simulink model "ASSIGNMENT1V6"  (R2020a)
settings: Solver=FixedStepAuto  StartTime=0.0  StopTime=5.0  FixedStep=1e-3  RelTol=1e-3  EnableMultiTasking=on
undefined symbols (not defined in the file): A0, A1, A3, A4, D0, D1, D10, D11, D12, D13, D2, D3, D4, D5, D6, D7, D8, D9, PTA0, PTA1, PTA2, PTB11, PTB2, PTB23, PTB3, PTB9, PTC11, PTC16, PTC17, PTC2, PTC3, PTC4, PTD0, PTD1, PTD2, PTD3
libraries: frdmk64flib x21
settings Model: ExtModeTrigDuration=5  Creator=Daniyal  LastModifiedBy=Daniyal
settings OptimizationCC: EnhancedBackFolding=on  PassReuseOutputArgsAs=Individual arguments  ZeroExternalMemoryAtStartup=off  ZeroInternalMemoryAtStartup=off  MaxStackSize=64  OptimizeBlockOrder=speed  DifferentSizesBufferReuse=on  OptimizationCustomize=off  EfficientTunableParamExpr=on
settings DebuggingCC: ParameterTunabilityLossMsg=error
settings HardwareCC: ProdBitPerPointer=32  ProdBitPerSizeT=32  ProdBitPerPtrDiffT=32  ProdLargestAtomicInteger=Long  ProdLargestAtomicFloat=Double  ProdWordSize=32  ProdHWDeviceType=ARM Compatible->ARM Cortex
settings SFSimCC: MATLABDynamicMemAlloc=off
settings RTWCC: SystemTargetFile=ert.tlc  HardwareBoard=NXP FRDM-K64F  TemplateMakefile=ert_default_tmf  Toolchain=GNU Tools for ARM Embedded Processors
settings CodeAppCC: ForceParamTrailComments=on  IgnoreCustomStorageClasses=off  OperatorAnnotations=on  SimulinkDataObjDesc=on  SFDataObjDesc=on  InsertBlockDesc=on

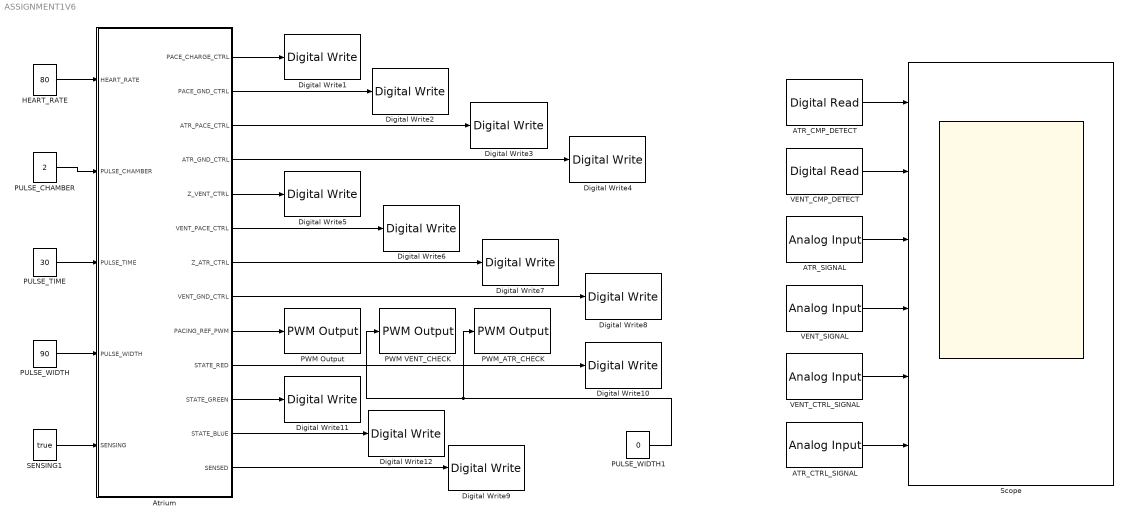
== system ASSIGNMENT1V6 ==
  ATR_CMP_DETECT : frdmk64flib/Digital Read  Whichpin=PTC16 (D0)  SampleTime=-1
  ATR_CTRL_SIGNAL : frdmk64flib/Analog Input  Whichpin=PTB11 (A3)  SampleTime=-1
  ATR_SIGNAL : frdmk64flib/Analog Input  Whichpin=PTB2 (A0)  SampleTime=-1
  Atrium : Stateflow chart  TreatAsAtomicUnit=on
  Digital Write1 : frdmk64flib/Digital Write  Whichpin=PTB9 (D2)
  Digital Write10 : frdmk64flib/Digital Write  Whichpin=RED_LED
  Digital Write11 : frdmk64flib/Digital Write  Whichpin=GREEN_LED
  Digital Write12 : frdmk64flib/Digital Write  Whichpin=BLUE_LED
  Digital Write2 : frdmk64flib/Digital Write  Whichpin=PTD0 (D10)
  Digital Write3 : frdmk64flib/Digital Write  Whichpin=PTA0 (D8)
  Digital Write4 : frdmk64flib/Digital Write  Whichpin=PTD2 (D11)
  Digital Write5 : frdmk64flib/Digital Write  Whichpin=PTC3 (D7)
  Digital Write6 : frdmk64flib/Digital Write  Whichpin=PTC4 (D9)
  Digital Write7 : frdmk64flib/Digital Write  Whichpin=PTB23 (D4)
  Digital Write8 : frdmk64flib/Digital Write  Whichpin=PTD3 (D12)
  Digital Write9 : frdmk64flib/Digital Write  Whichpin=PTD1 (D13)
  HEART_RATE : Constant  Value=80
  PULSE_CHAMBER : Constant  Value=2
  PULSE_TIME : Constant  Value=30
  PULSE_WIDTH : Constant  Value=90
  PULSE_WIDTH1 : Constant  Value=0
  PWM Output : frdmk64flib/PWM Output  Whichpin=PTA2 (D5)  InitialFrequency=2000  InitialDutyCycle=70
  PWM VENT_CHECK : frdmk64flib/PWM Output  Whichpin=PTA1 (D3)  InitialFrequency=2000  InitialDutyCycle=80
  PWM_ATR_CHECK : frdmk64flib/PWM Output  Whichpin=PTC2 (D6)  InitialFrequency=2000  InitialDutyCycle=0
  SENSING1 : Constant  Value=true  OutDataTypeStr=boolean
  Scope : Scope  NumInputPorts=6
  VENT_CMP_DETECT : frdmk64flib/Digital Read  Whichpin=PTC17 (D1)  SampleTime=-1
  VENT_CTRL_SIGNAL : frdmk64flib/Analog Input  Whichpin=PTC11 (A4)  SampleTime=-1
  VENT_SIGNAL : frdmk64flib/Analog Input  Whichpin=PTB3 (A1)  SampleTime=-1
  wires:
  Atrium/4(ATR_GND_CTRL) -> Digital Write4/1
  Atrium/5(Z_VENT_CTRL) -> Digital Write5/1
  Atrium/6(VENT_PACE_CTRL) -> Digital Write6/1
  Atrium/3(ATR_PACE_CTRL) -> Digital Write3/1
  Atrium/8(VENT_GND_CTRL) -> Digital Write8/1
  Atrium/10(STATE_RED) -> Digital Write10/1
  Atrium/11(STATE_GREEN) -> Digital Write11/1
  Atrium/12(STATE_BLUE) -> Digital Write12/1
  Atrium/1(PACE_CHARGE_CTRL) -> Digital Write1/1
  HEART_RATE/1 -> Atrium/1(HEART_RATE)
  Atrium/7(Z_ATR_CTRL) -> Digital Write7/1
  PULSE_WIDTH/1 -> Atrium/4(PULSE_WIDTH)
  Atrium/2(PACE_GND_CTRL) -> Digital Write2/1
  PULSE_CHAMBER/1 -> Atrium/2(PULSE_CHAMBER)
  PULSE_TIME/1 -> Atrium/3(PULSE_TIME)
  SENSING1/1 -> Atrium/5(SENSING)
  Atrium/13(SENSED) -> Digital Write9/1
  ATR_CMP_DETECT/1 -> Scope/1
  ATR_SIGNAL/1 -> Scope/3
  VENT_SIGNAL/1 -> Scope/4
  VENT_CTRL_SIGNAL/1 -> Scope/5
  ATR_CTRL_SIGNAL/1 -> Scope/6
  VENT_CMP_DETECT/1 -> Scope/2
  Atrium/9(PACING_REF_PWM) -> PWM Output/1
  PULSE_WIDTH1/1 -> PWM_ATR_CHECK/1, PWM VENT_CHECK/1

== stateflow chart ASSIGNMENT1V6/Atrium ==
  state PULSE_ATRIUM
    entry:
    during:
    SENSED = SENSING;
    STATE_RED = 0;
    STATE_GREEN = 0;
    STATE_BLUE = 1;
    PACE_CHARGE_CTRL =  false;
    PACE_GND_CTRL = true;
    ATR_PACE_CTRL = true;
    ATR_GND_CTRL =  false;
    Z_ATR_CTRL = false;
    Z_VENT_CTRL =  false;
    VENT_GND_CTRL =false;
    VENT_PACE_CTRL =  false;
    exit:
  state CHARGE
    entry:
    during:
    SENSED = SENSING;
    STATE_RED = 1;
    STATE_GREEN = 0;
    STATE_BLUE = 0;
    ATR_PACE_CTRL = false;
    VENT_PACE_CTRL  = false;
    PACING_REF_PWM = PULSE_WIDTH;
    PACE_CHARGE_CTRL = true;
    PACE_GND_CTRL = true;
    VENT_PACE_CTRL = false;
    Z_ATR_CTRL =  false;
    Z_VENT_CTRL =  false;
    ATR_PACE_CTRL =  false;
    if (PULSE_CHAMBER==1)
    ATR_GND_CTRL = true;
    VENT_GND_CTRL =  false;
    else
    ATR_GND_CTRL = false;
    VENT_GND_CTRL = true;
    end
    exit:
  state PULSE_VENTRICLE
    entry:
    during:
    SENSED = SENSING;
    STATE_RED = 0;
    STATE_GREEN = 1;
    STATE_BLUE = 0;
    PACE_CHARGE_CTRL =  false;
    PACE_GND_CTRL = true;
    ATR_PACE_CTRL = false;
    ATR_GND_CTRL =  false;
    Z_ATR_CTRL = false;
    Z_VENT_CTRL =  false;
    VENT_GND_CTRL =false;
    VENT_PACE_CTRL =  true;
    exit:
  CHARGE -> PULSE_ATRIUM [order 1] : [[after((60000/HEART_RATE)-PULSE_TIME,msec) & (PULSE_CHAMBER==1) ]]
  (default) -> CHARGE
  PULSE_ATRIUM -> CHARGE : [after(PULSE_TIME,msec)]
  PULSE_VENTRICLE -> CHARGE : [after(PULSE_TIME,msec)]
  CHARGE -> PULSE_VENTRICLE [order 2] : [[after((60000/HEART_RATE)-PULSE_TIME,msec) & (PULSE_CHAMBER==2) ]]
  data: HEART_RATE input double; PULSE_CHAMBER input double; PULSE_TIME input double; PULSE_WIDTH input double; PACE_CHARGE_CTRL output boolean =false; PACE_GND_CTRL output boolean =false; ATR_PACE_CTRL output boolean =false; ATR_GND_CTRL output boolean =false; Z_VENT_CTRL output boolean =false; VENT_PACE_CTRL output boolean =false; Z_ATR_CTRL output boolean =false; VENT_GND_CTRL output boolean =false; PACING_REF_PWM output double; STATE_RED output int16; STATE_GREEN output int16; STATE_BLUE output int16; SENSING input boolean; SENSED output
